simulink model "testing_project"  (R2024b)
settings: Solver=VariableStepAuto  StartTime=0.0  StopTime=10  RelTol=1e-3
undefined symbols (not defined in the file or in its folder): Ion, Lithium
libraries: fuzblock x1, spsBatteryLib x1, spsControlledCurrentSourceLib x1, sps_lib x1
settings Model: Creator=Naveen  LastModifiedBy=Naveen

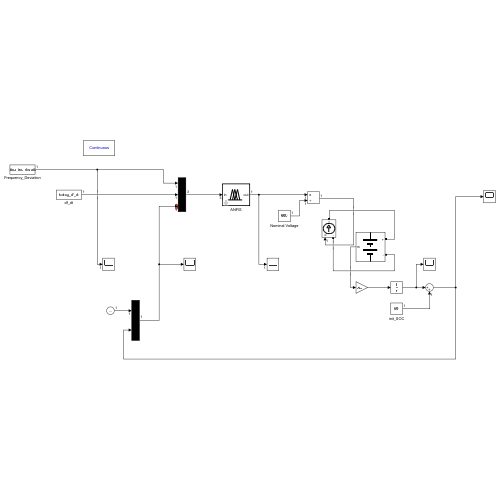
[thumbnail: Simulink's stored preview of the top-level diagram]
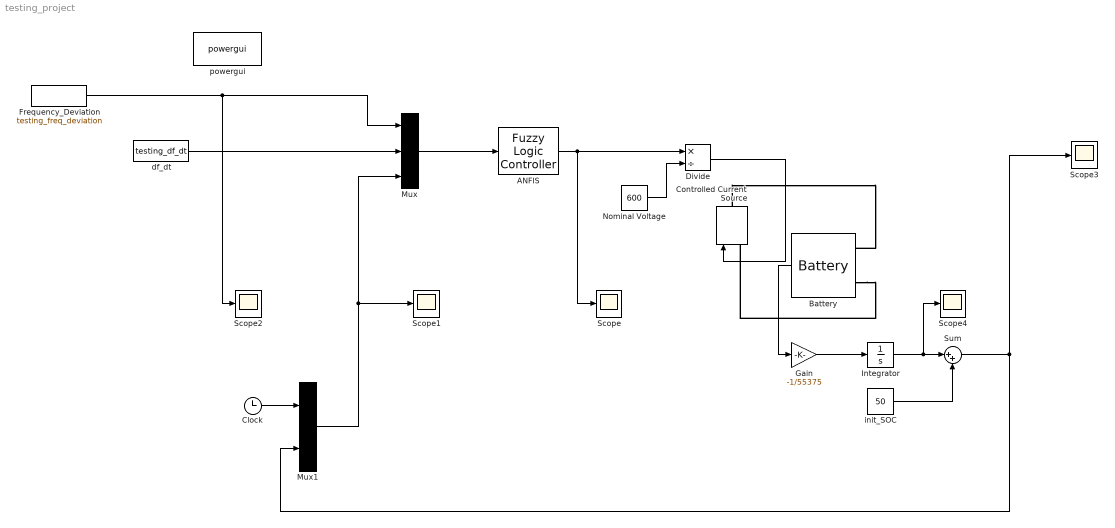
== system testing_project ==
  ANFIS : fuzblock/Fuzzy Logic  Controller  FIS='pfnn_trained.fis'  OutputSampleNumber=101  DataType=double  FuzzifiedInputs=off  RuleFiringStrengths=off  RuleOutputs=off  AggregatedOutputs=off  SimulateUsing=Interpreted execution  OutOfRangeInputValueMessage=warning  NoRuleFiredMessage=warning  EmptyOutputFuzzySetMessage=warning
  Battery : spsBatteryLib/Battery  BatType=Lithium-Ion  NomV=600  NomQ=55375  SOC=50  Batt_Tr=30  PresetModel=on  MaxQ=55375  MinV=450  FullV=698.3923  Dis_rate=24076.087  R=0.00010835  Normal_OP=50078.2609  expZone="[648.23151      2720.5978]"
  Clock : Clock
  Controlled Current Source : spsControlledCurrentSourceLib/Controlled Current Source  Initialize=on  Source_Type=AC  Amplitude=0  Phase=0  Frequency=0  Measurements=None
  Divide : Product  Inputs=*/
  Frequency_Deviation : FromWorkspace  VariableName=testing_freq_deviation
  Gain : Gain  Gain=-1/55375
  Integrator : Integrator
  Mux : Mux  Inputs=3
  Mux1 : Mux  Inputs=2
  Nominal Voltage : Constant  Value=600
  Scope{,1..4} (5 alike) : Scope
  Sum : Sum  Inputs=|++
  df_dt : FromWorkspace  VariableName=testing_df_dt
  init_SOC : Constant  Value=50
  powergui : sps_lib/powergui  Priority=1  SimulationMode=Continuous  SampleTime=50e-6  frequency=60  Iterations=50  frequencyindice=0  Pbase=100e6  ErrMax=1e-4  UnitsV=kV  UnitsW=MW  buscounter=0  FunctionMessages=off  echomessages=off  EnableUseOfTLC=off  CurrentSourceSwitches=off  DisableSnubberDevices=off  DisableRonSwitches=off  DisableVfSwitches=off  DisplayEquations=off  AutomaticDiscreteSolvers=off  SolverType=Tustin/Backward Euler (TBE)  Interpol=off  ExternalGateDelay=off  methode=off  Ts=100  x0status=blocks  SPID=on  SwTol=0  HookPort=off  NonlinearTolerance=1e-4  nMaxIteration=100  ContinueOnMaxIteration=off  RestoreLinks=warning  ResistiveCurrentMeasurement=off  Frange=[0:2:500]  Ylog=off  Xlog=on  ShowGrid=off  save=off  variable=ZData  structure=0  ZoomFFT=off  StartTime=0.0  cycles=1  DisplayStyle=1  fundamental=60  FreqAxis=off  MaxFrequency=1000  frequencyindicesteady=1  RmsSteady=1  display=off
  wires:
  Mux/1 -> ANFIS/1
  Frequency_Deviation/1 -> Scope2/1, Mux/1
  df_dt/1 -> Mux/2
  Sum/1 -> Scope3/1, Mux1/2
  ANFIS/1 -> Divide/1, Scope/1
  Nominal Voltage/1 -> Divide/2
  Divide/1 -> Controlled Current Source/1
  Battery/1 -> Gain/1
  Gain/1 -> Integrator/1
  Integrator/1 -> Scope4/1, Sum/1
  init_SOC/1 -> Sum/2
  Clock/1 -> Mux1/1
  Mux1/1 -> Scope1/1, Mux/3
  connections:
  Controlled Current Source/RConn1 -- Battery/LConn1
  Battery/LConn2 -- Controlled Current Source/LConn1
